simulink model "ESTS_VVSO_test"  (R2023b)
settings: Solver=VariableStepAuto  StartTime=0.0  StopTime=10.0  RelTol=1e-3
libraries: simulink x1, ESTS_VVSO x1
settings Model: Creator=blatak  LastModifiedBy=blatak

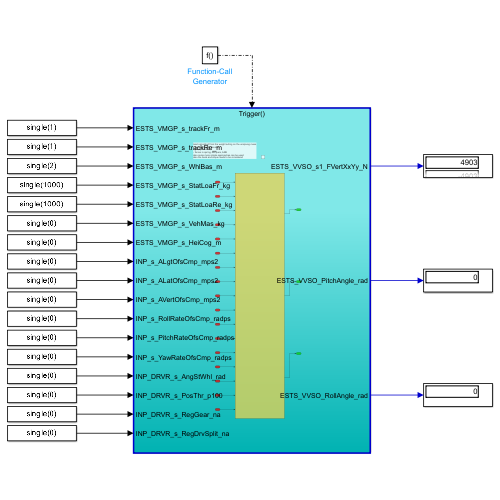
[thumbnail: Simulink's stored preview of the top-level diagram]
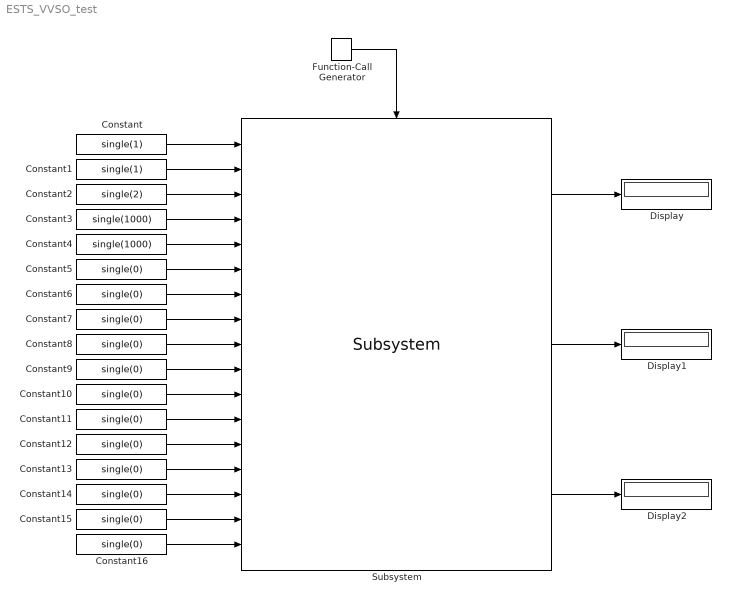
== system ESTS_VVSO_test ==
  Constant : Constant  Value=single(1)
  Constant1 : Constant  Value=single(1)
  Constant{5..16} (12 alike) : Constant  Value=single(0)
  Constant2 : Constant  Value=single(2)
  Constant3 : Constant  Value=single(1000)
  Constant4 : Constant  Value=single(1000)
  Display : Display
  Display1 : Display
  Display2 : Display
  Function-Call Generator : simulink/Ports & Subsystems/Function-Call Generator  sample_time=0.01  numberOfIterations=1  DisallowWideOutput=off
  Subsystem : ESTS_VVSO/Subsystem  SystemSampleTime=-1  VariantActivationTime=update diagram  AllowFlexibleInterface=on  Latency=0  AutoFrameSizeCalculation=off
  wires:
  Function-Call Generator/1 -> Subsystem/Trigger
  Subsystem/1 -> Display/1
  Subsystem/2 -> Display1/1
  Subsystem/3 -> Display2/1
  Constant/1 -> Subsystem/1
  Constant1/1 -> Subsystem/2
  Constant2/1 -> Subsystem/3
  Constant3/1 -> Subsystem/4
  Constant4/1 -> Subsystem/5
  Constant5/1 -> Subsystem/6
  Constant6/1 -> Subsystem/7
  Constant7/1 -> Subsystem/8
  Constant8/1 -> Subsystem/9
  Constant9/1 -> Subsystem/10
  Constant10/1 -> Subsystem/11
  Constant11/1 -> Subsystem/12
  Constant12/1 -> Subsystem/13
  Constant13/1 -> Subsystem/14
  Constant14/1 -> Subsystem/15
  Constant15/1 -> Subsystem/16
  Constant16/1 -> Subsystem/17
